simulink model "model_VS_PSH"  (R2020b)
settings: Solver=ode1  StartTime=0.0  StopTime=60  RelTol=1e-3
InitFcn:
  | xInitial = init_power_wind_dfig_det;
  | %Ts=5e-6;
values from neighbouring files (symbols this model uses):
  Cap_DClink = 20000e-6    (= 0.02)    [MAIN_VS_PSH.m]
  Efficiency = 0.9    [MAIN_VS_PSH.m]
  Fnom = 60    [MAIN_VS_PSH.m]
  H = 2.7    [MAIN_VS_PSH.m]
  Initial_Head = 1    [MAIN_VS_PSH.m]
  Initial_SOC = 0.8    [MAIN_VS_PSH.m]
  kmVdc = 20e3    (= 20000)    [MAIN_VS_PSH.m]
  Kp = 1    [MAIN_VS_PSH.m]
  kp_pll = 0.236583    [MAIN_T_PSH_IEEE39.m]    (also in MAIN_VS_PSH.m)
  Kpg = 1.3466e-5    (= 1.3466e-05)    [MAIN_VS_PSH.m]
  Kpr = 4.559e-5    (= 4.559e-05)    [MAIN_VS_PSH.m]
  Kvp = 6.1584    [MAIN_VS_PSH.m]
  Lm = Lb*Lmpu    [MAIN_VS_PSH.m]
  Lph = 3e-4    (= 0.0003)    [MAIN_VS_PSH.m]
  Lr = Lb*Lrpu    [MAIN_VS_PSH.m]
  Lrleakpu = 0.11    [MAIN_VS_PSH.m]
  Ls = Lb*Lspu    [MAIN_VS_PSH.m]
  Lsleakpu = 0.102    [MAIN_VS_PSH.m]
  Max_discharge_hrs = 10    [MAIN_VS_PSH.m]
  Mode = 0    [MAIN_FS_PSH_IEEE39.m]    (also in MAIN_VS_PSH.m = 1; plots_FS_PSH_IEEE39.m = 1; plots_VS_PSH.m = 1)
  Pnom = Srated*1e6    (= 300000000)    [MAIN_VS_PSH.m]
  Pref = 0.9    [MAIN_T_PSH_IEEE39.m]    (also in MAIN_VS_PSH.m = 1)
  QnL = 0    [MAIN_VS_PSH.m]
  Qref = 0    [MAIN_VS_PSH.m]
  Rrpu = 0.00607    [MAIN_VS_PSH.m]
  Rspu = 0.0054    [MAIN_VS_PSH.m]
  sigma = 1- Lmpu*Lmpu/(Lrpu^2)    (= 0.0485899542692)    [MAIN_VS_PSH.m]
  Srated = 300    [MAIN_VS_PSH.m]
  t_sw_off = 220    [MAIN_FS_PSH_IEEE39.m]    (also in MAIN_T_PSH_IEEE39.m; MAIN_VS_PSH.m = 45)
  t_sw_on = 130    [MAIN_FS_PSH_IEEE39.m]    (also in MAIN_T_PSH_IEEE39.m; MAIN_VS_PSH.m = 35)
  Ti = 0.01    [MAIN_VS_PSH.m]
  ti_pll = 0.0224242    [MAIN_T_PSH_IEEE39.m]    (also in MAIN_VS_PSH.m)
  Tig = 59.0944    [MAIN_VS_PSH.m]
  Tir = 197.953    [MAIN_VS_PSH.m]
  Ts = 25e-6    (= 2.5e-05)    [MAIN_FS_PSH_IEEE39.m]    (also in MAIN_T_PSH_IEEE39.m; MAIN_VS_PSH.m = 1e-07)
  TurnsRatio = 0.37912    [MAIN_VS_PSH.m]
  Tvi = 0.0013532    [MAIN_VS_PSH.m]
  V1 = sqrt(2)*Vnom_grid/sqrt(3)    [MAIN_VS_PSH.m]
  Vdc_ref = 40e3    (= 40000)    [MAIN_VS_PSH.m]
  Vnom_grid = 18e3    (= 18000)    [MAIN_VS_PSH.m]
  W1 = 2*pi*Fnom    (= 376.991118431)    [MAIN_VS_PSH.m]
  Xph = Lph*W1    (= 0.113097335529)    [MAIN_VS_PSH.m]
undefined symbols (not defined in the file or in its folder): magnitude
libraries: powerlib x49, powerlib_meascontrol x21, pid_lib x10, simulink_extras x4, simulink x1
(part 1 of 3)
settings Model: FPTRunName=Active  SimulationMode=accelerator  ExtModeAutoUpdateStatusClock=off  Creator=MathWorks  LastModifiedBy=mjimene
settings DataIOCC: MaxDataPoints=1500  SaveFormat=StructureWithTime  SignalLoggingSaveFormat=ModelDataLogs  SaveOutput=off  SignalLogging=off  DSMLogging=off  SaveTime=off
settings OptimizationCC: ExpressionDepthLimit=2147483647  InitFltsAndDblsToZero=on  LifeSpan=inf
settings DebuggingCC: SaveWithParameterizedLinksMsg=none  UnderspecifiedInitializationDetection=Classic  MergeDetectMultiDrivingBlocksExec=none  SignalResolutionControl=TryResolveAllWithWarning  SolverPrmCheckMsg=warning  FcnCallInpInsideContextMsg=warning  UnconnectedLineMsg=none  StateNameClashWarn=warning  SFUnexpectedBacktrackingDiag=warning  SFNoUnconditionalDefaultTransitionDiag=warning  SFExecutionAtInitializationDiag=none  ArithmeticOperatorsInVariantConditions=warning
settings HardwareCC: ProdBitPerPointer=32  ProdBitPerSizeT=32  ProdBitPerPtrDiffT=32  ProdLargestAtomicFloat=None  ProdIntDivRoundTo=Undefined  ProdEndianess=Unspecified  ProdWordSize=32  ProdHWDeviceType=32-bit Generic
settings ModelReferenceCC: PropagateSignalLabelsOutOfModel=off
settings SFSimCC: SimUseLocalCustomCode=off  CustomCodeUndefinedFunction=UseInterfaceOnly
settings RTWCC: RTWUseLocalCustomCode=off
settings CodeAppCC: StateflowObjectComments=on
settings GRTTargetCC: TargetFcnLib=ansi_tfl_tmw.mat  TargetLangStandard=C89/C90 (ANSI)  CombineOutputUpdateFcns=off  GRTInterface=on
settings ConfigComp: CovMetricSettings=dw  CovSaveCumulativeToWorkspaceVar=on  CovSaveSingleToWorkspaceVar=on  CovExternalEMLEnable=off  CovSFcnEnable=off
settings SimscapeCC: SimscapeNormalizeSystem=off

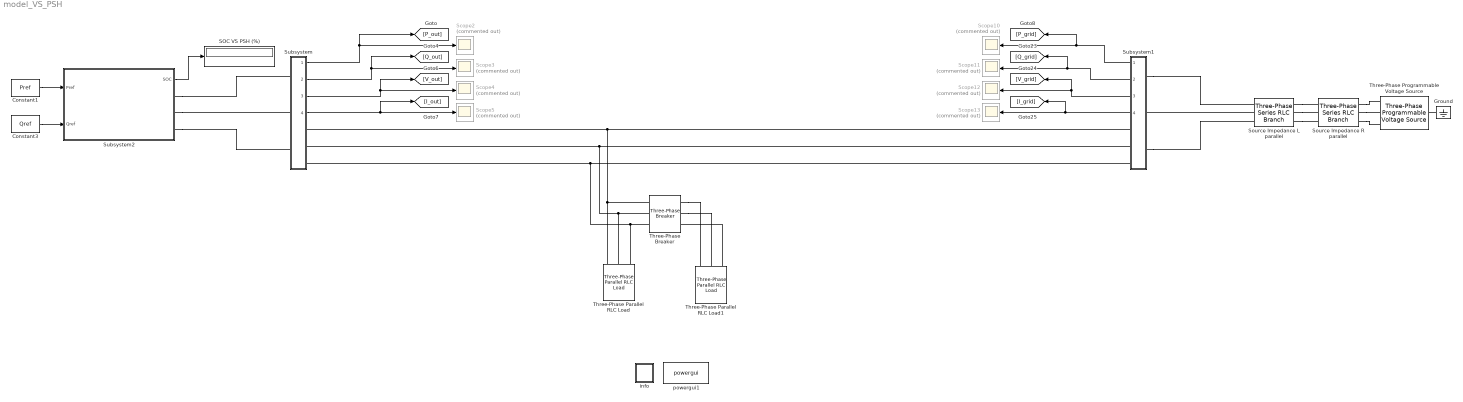
== system model_VS_PSH ==
  Constant1 : Constant  Value=Pref
  Constant3 : Constant  Value=Qref
  Ground : powerlib/Elements/Ground  LConnTagsString=a
  SOC VS PSH (%) : Display
  Scope{2..5,10..13} (8 alike) : Scope  Commented=on
  Source Impedance R parallel : powerlib/Elements/Three-Phase Series RLC Branch  LConnTagsString=A|B|C  RConnTagsString=A|B|C  BranchType=R  Resistance=0.0945*0.1/490  Inductance=0.01  Capacitance=[]  Measurements=None
  Source Impedance L parallel : powerlib/Elements/Three-Phase Series RLC Branch  LConnTagsString=A|B|C  RConnTagsString=A|B|C  BranchType=L  Resistance=1  Inductance=14.2e-4/490  Capacitance=[]  Measurements=None
  Subsystem : Subsystem
  Subsystem1 : Subsystem
  Subsystem2 : Subsystem
  Three-Phase Parallel RLC Load : powerlib/Elements/Three-Phase Parallel RLC Load  LConnTagsString=A|B|C  Configuration=Y (grounded)  NominalVoltage=18e3  Vabc=[1e3 1e3 1e3]  Vabcp=[1e3 1e3 1e3]  NominalFrequency=60  UnbalancedPower=off  ActivePower=50e6  InductivePower=0  CapacitivePower=0  Pabc=[10e3 9e3 11e3]  QLabc=[100 90 110]  QCabc=[100 90 110]  Pabcp=[10e3 9e3 11e3]  QLabcp=[100 90 110]  QCabcp=[100 90 110]  Measurements=None  LoadType=constant Z
  Three-Phase Parallel RLC Load1 : powerlib/Elements/Three-Phase Parallel RLC Load  LConnTagsString=A|B|C  Configuration=Y (grounded)  NominalVoltage=18e3  Vabc=[1e3 1e3 1e3]  Vabcp=[1e3 1e3 1e3]  NominalFrequency=60  UnbalancedPower=off  ActivePower=50e6  InductivePower=0  CapacitivePower=0  Pabc=[10e3 9e3 11e3]  QLabc=[100 90 110]  QCabc=[100 90 110]  Pabcp=[10e3 9e3 11e3]  QLabcp=[100 90 110]  QCabcp=[100 90 110]  Measurements=None  LoadType=constant Z
  Three-Phase Programmable Voltage Source : powerlib/Electrical Sources/Three-Phase Programmable Voltage Source  PositiveSequence=[18e3 0 60]  VariationEntity=None  VariationType=Table of time-amplitude pairs  VariationTypeAlt=Step  VariationStep=-0.5  VariationRate=10  VariationMagnitude=0.3  VariationFrequency=2  VariationTiming=[30 37]  VariationPhaseA=off  Amplitudes=[1 0.8 1.2 1.0]  TimeValues=[0 0.1 0.15 0.2]  HarmonicGeneration=off  HarmonicA=[3 0.2 -25 0]  HarmonicB=[2 0.15 35 2]  Timing="[0.05  3]"  BusType=swing  Pref=0  Qref=0  Qmin=-inf  Qmax=inf
  Three-Phase Breaker : powerlib/Elements/Three-Phase Breaker  InitialState=open  SwitchA=on  SwitchB=on  SwitchC=on  SwitchTimes=[t_sw_on t_sw_off]  External=off  BreakerResistance=0.01  SnubberResistance=1e6  SnubberCapacitance=inf  Measurements=None
  info : Subsystem
      settings: OpenFcn=showdemo(bdroot(gcb))
      mask Display: disp('?')
  powergui1 : powerlib/powergui  Priority=1  SimulationMode=Discrete  SampleTime=Ts  frequency=60  Iterations=50  frequencyindice=0  Pbase=100e6  ErrMax=1e-4  UnitsV=kV  UnitsW=MW  buscounter=0  FunctionMessages=off  echomessages=off  EnableUseOfTLC=off  CurrentSourceSwitches=off  DisableSnubberDevices=off  DisableRonSwitches=off  DisableVfSwitches=off  DisplayEquations=off  AutomaticDiscreteSolvers=off  SolverType=Tustin/Backward Euler (TBE)  Interpol=off  ExternalGateDelay=off  methode=off  Ts=100  x0status=blocks  SPID=on  SwTol=0  HookPort=off  NonlinearTolerance=1e-4  nMaxIteration=100  ContinueOnMaxIteration=off  RestoreLinks=warning  ResistiveCurrentMeasurement=off  Frange=[0:2:500]  Ylog=off  Xlog=on  ShowGrid=off  save=off  variable=ZData  structure=0  ZoomFFT=off  StartTime=0.0  cycles=1  DisplayStyle=1  fundamental=60  FreqAxis=off  MaxFrequency=1000  frequencyindicesteady=1  RmsSteady=1  display=off
  wires:
  Subsystem/1(Out1) -> [P_out], Scope2/1
  Subsystem/2(Out2) -> [Q_out], Scope3/1
  Subsystem/3(Out3) -> [V_out], Scope4/1
  Subsystem/4(Out4) -> [I_out], Scope5/1
  Subsystem1/4(Out4) -> [I_grid], Scope13/1
  Subsystem1/3(Out3) -> [V_grid], Scope12/1
  Subsystem1/2(Out2) -> [Q_grid], Scope11/1
  Subsystem1/1(Out1) -> [P_grid], Scope10/1
  Constant1/1 -> Subsystem2/1(Pref)
  Constant3/1 -> Subsystem2/2(Qref)
  Subsystem2/1(SOC) -> SOC VS PSH (%)/1
  connections:
  Three-Phase Parallel RLC Load1/LConn3 -- Three-Phase Breaker/RConn3
  Three-Phase Breaker/RConn2 -- Three-Phase Parallel RLC Load1/LConn2
  Three-Phase Breaker/RConn1 -- Three-Phase Parallel RLC Load1/LConn1
  Subsystem/RConn1 -- Three-Phase Parallel RLC Load/LConn1 -- Three-Phase Breaker/LConn1 -- Subsystem1/RConn1
  Subsystem1/RConn2 -- Three-Phase Parallel RLC Load/LConn2 -- Three-Phase Breaker/LConn2 -- Subsystem/RConn2
  Three-Phase Parallel RLC Load/LConn3 -- Three-Phase Breaker/LConn3 -- Subsystem1/RConn3 -- Subsystem/RConn3
  Subsystem2/RConn1 -- Subsystem/LConn1
  Subsystem2/RConn2 -- Subsystem/LConn2
  Subsystem2/RConn3 -- Subsystem/LConn3
  Subsystem1/LConn1 -- Source Impedance L parallel/LConn1
  Source Impedance L parallel/LConn2 -- Subsystem1/LConn2
  Subsystem1/LConn3 -- Source Impedance L parallel/LConn3
  Ground/LConn1 -- Three-Phase Programmable Voltage Source/LConn1
  Source Impedance L parallel/RConn1 -- Source Impedance R parallel/LConn1
  Source Impedance L parallel/RConn2 -- Source Impedance R parallel/LConn2
  Source Impedance L parallel/RConn3 -- Source Impedance R parallel/LConn3
  Source Impedance R parallel/RConn1 -- Three-Phase Programmable Voltage Source/RConn1
  Source Impedance R parallel/RConn2 -- Three-Phase Programmable Voltage Source/RConn2
  Source Impedance R parallel/RConn3 -- Three-Phase Programmable Voltage Source/RConn3

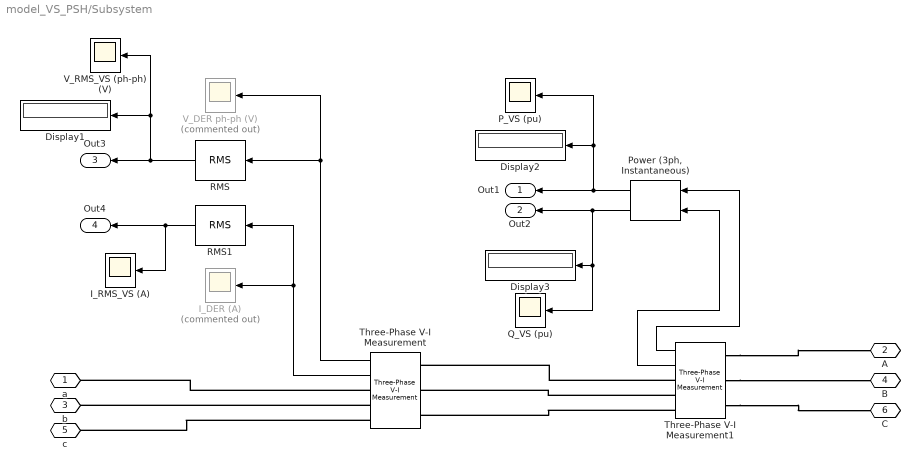
== system model_VS_PSH/Subsystem ==
  Display1 : Display
  Display2 : Display
  Display3 : Display
  I_DER (A) : Scope  Commented=on
  I_RMS_VS (A) : Scope
  P_VS (pu) : Scope
  "Power (3ph, Instantaneous)" : powerlib_meascontrol/Measurements/Power (3ph, Instantaneous)
  Q_VS (pu) : Scope
  RMS : powerlib_meascontrol/Measurements/RMS  TrueRMS=off  Freq=60  RMSInit=1  Ts=Ts
  RMS1 : powerlib_meascontrol/Measurements/RMS  TrueRMS=off  Freq=60  RMSInit=1  Ts=Ts
  Three-Phase V-I Measurement : powerlib/Measurements/Three-Phase V-I Measurement  VoltageMeasurement=phase-to-phase  SetLabelV=off  LabelV=Vabc  Vpu=off  VpuLL=off  CurrentMeasurement=yes  SetLabelI=off  LabelI=Iabc  Ipu=off  Pbase=100e6  Vbase=500e3  OutputType=Complex  PhasorSimulation=off  PSBequivalent=0
  Three-Phase V-I Measurement1 : powerlib/Measurements/Three-Phase V-I Measurement  VoltageMeasurement=phase-to-ground  SetLabelV=off  LabelV=Vabc  Vpu=off  VpuLL=off  CurrentMeasurement=yes  SetLabelI=off  LabelI=Iabc  Ipu=off  Pbase=100e6  Vbase=500e3  OutputType=Complex  PhasorSimulation=off  PSBequivalent=0
  V_DER ph-ph (V) : Scope  Commented=on
  V_RMS_VS (ph-ph) (V) : Scope
  a : PMIOPort  Side=Right
  A : PMIOPort  Port=2  Side=Left
  b : PMIOPort  Port=3  Side=Right
  B : PMIOPort  Port=4  Side=Left
  c : PMIOPort  Port=5  Side=Right
  C : PMIOPort  Port=6  Side=Left
  Out1 : Outport
  Out2 : Outport  Port=2
  Out3 : Outport  Port=3
  Out4 : Outport  Port=4
  wires:
  Three-Phase V-I Measurement1/1 -> "Power (3ph, Instantaneous)"/1
  Three-Phase V-I Measurement/1 -> RMS/1, V_DER ph-ph (V)/1
  Three-Phase V-I Measurement/2 -> RMS1/1, I_DER (A)/1
  RMS1/1 -> Out4/1, I_RMS_VS (A)/1
  Three-Phase V-I Measurement1/2 -> "Power (3ph, Instantaneous)"/2
  RMS/1 -> Out3/1, V_RMS_VS (ph-ph) (V)/1, Display1/1
  "Power (3ph, Instantaneous)"/1 -> Display2/1, P_VS (pu)/1, Out1/1
  "Power (3ph, Instantaneous)"/2 -> Q_VS (pu)/1, Display3/1, Out2/1
  connections:
  Three-Phase V-I Measurement1/RConn1 -- Three-Phase V-I Measurement/LConn1
  Three-Phase V-I Measurement1/RConn2 -- Three-Phase V-I Measurement/LConn2
  Three-Phase V-I Measurement1/RConn3 -- Three-Phase V-I Measurement/LConn3
  Three-Phase V-I Measurement/RConn2 -- b/RConn1
  Three-Phase V-I Measurement/RConn3 -- c/RConn1
  Three-Phase V-I Measurement1/LConn1 -- A/RConn1
  Three-Phase V-I Measurement/RConn1 -- a/RConn1
  Three-Phase V-I Measurement1/LConn2 -- B/RConn1
  Three-Phase V-I Measurement1/LConn3 -- C/RConn1

== system model_VS_PSH/Subsystem1 ==
  "Power (3ph, Instantaneous)" : powerlib_meascontrol/Measurements/Power (3ph, Instantaneous)
  Three-Phase V-I Measurement : powerlib/Measurements/Three-Phase V-I Measurement  VoltageMeasurement=phase-to-phase  SetLabelV=off  LabelV=Vabc  Vpu=off  VpuLL=off  CurrentMeasurement=yes  SetLabelI=off  LabelI=Iabc  Ipu=off  Pbase=100e6  Vbase=500e3  OutputType=Complex  PhasorSimulation=off  PSBequivalent=0
  Three-Phase V-I Measurement1 : powerlib/Measurements/Three-Phase V-I Measurement  VoltageMeasurement=phase-to-ground  SetLabelV=off  LabelV=Vabc  Vpu=off  VpuLL=off  CurrentMeasurement=yes  SetLabelI=off  LabelI=Iabc  Ipu=off  Pbase=100e6  Vbase=500e3  OutputType=Complex  PhasorSimulation=off  PSBequivalent=0
  a : PMIOPort  Side=Right
  A : PMIOPort  Port=2  Side=Left
  b : PMIOPort  Port=3  Side=Right
  B : PMIOPort  Port=4  Side=Left
  c : PMIOPort  Port=5  Side=Right
  C : PMIOPort  Port=6  Side=Left
  Out1 : Outport
  Out2 : Outport  Port=2
  Out3 : Outport  Port=3
  Out4 : Outport  Port=4
  wires:
  Three-Phase V-I Measurement1/1 -> "Power (3ph, Instantaneous)"/1
  Three-Phase V-I Measurement/2 -> Out4/1
  Three-Phase V-I Measurement1/2 -> "Power (3ph, Instantaneous)"/2
  Three-Phase V-I Measurement/1 -> Out3/1
  "Power (3ph, Instantaneous)"/1 -> Out1/1
  "Power (3ph, Instantaneous)"/2 -> Out2/1
  connections:
  Three-Phase V-I Measurement1/RConn1 -- Three-Phase V-I Measurement/LConn1
  Three-Phase V-I Measurement1/RConn2 -- Three-Phase V-I Measurement/LConn2
  Three-Phase V-I Measurement1/RConn3 -- Three-Phase V-I Measurement/LConn3
  Three-Phase V-I Measurement/RConn2 -- b/RConn1
  Three-Phase V-I Measurement/RConn3 -- c/RConn1
  Three-Phase V-I Measurement1/LConn1 -- A/RConn1
  Three-Phase V-I Measurement/RConn1 -- a/RConn1
  Three-Phase V-I Measurement1/LConn2 -- B/RConn1
  Three-Phase V-I Measurement1/LConn3 -- C/RConn1

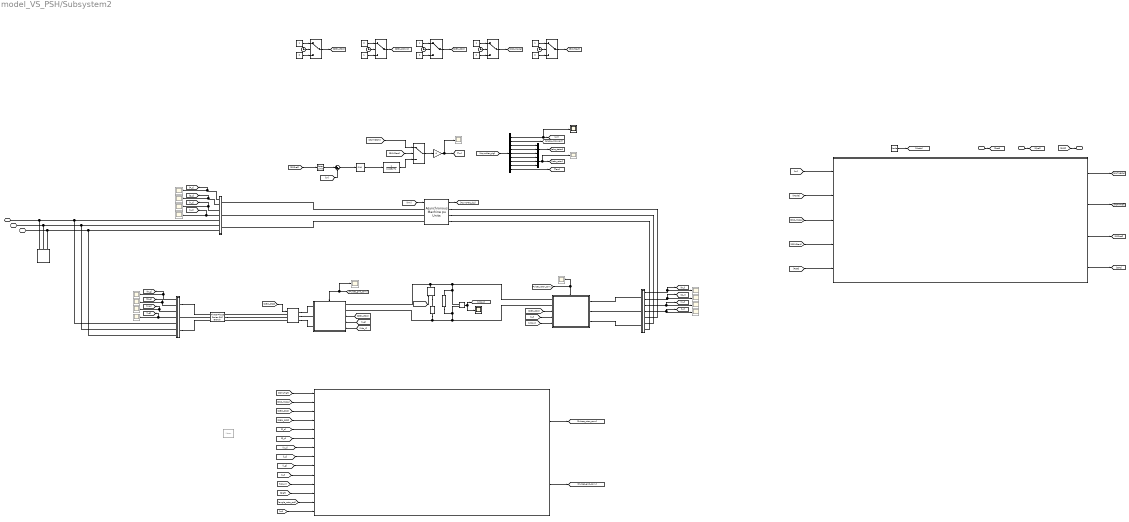
== system model_VS_PSH/Subsystem2 ==
  note: AC-DC-AC Converter
      | Average Model
  note: GSC measurements
  note: Variable Speed Hydro PSH
  note: RSC measurements
  note: Wound-Rotor
      | Induction Generator
  note: Measurement and controls
  note: Intialization sequence
  Pref : Inport
  Qref : Inport  Port=2
  Asynchronous Machine pu Units : powerlib/Machines/Asynchronous Machine pu Units  RotorType=Wound  PresetModel=No  MechanicalLoad=Torque Tm  ShowDetailedParameters=on  ReferenceFrame=Rotor  Units=pu  MeasurementBus=off  NominalParameters=[ Pnom Vnom_grid Fnom ]  Stator=[ Rspu Lsleakpu]  Rotor=[ Rrpu Lrleakpu]  Cage1=[0.01909 0.0397]  Cage2=[0.01909 0.0397]  Lm=Lmpu  Mechanical=[H 0.01 1]  PolePairs=3  InitialConditions=[0, pi, 0,0,0, 0,-120,120, 0,0,0, 0,-120, 120]  SimulateSaturation=off  Saturation="[0.212,0.4201,0.8125,1.0979,1.4799,2.2457,3.2586,4.5763,6.4763 ;   0.5,0.7,0.9,1,1.1,1.2 ,1.3,1.4,1.5]"  LoadFlowParameters=0  TsPowergui=0  TsBlock=-1  IterativeModel=Trapezoidal non iterative  IterativeDiscreteModel=Trapezoidal non iterative  Pmec=0
      settings: SourceProductBaseCode=PS
  Breaker1 : powerlib/Elements/Breaker  InitialState=1  SwitchingTimes="[1/60  5/60]"  External=on  BreakerResistance=0.01  SnubberResistance=1e6  SnubberCapacitance=inf  Measurements=None  MoreParameters=on  NoBreakLoop=off
  Bus Selector : BusSelector  OutputSignals=Mechanical.Rotor speed (wm),Mechanical.Rotor angle thetam (rad),Stator measurements.Stator current is_a (pu),Stator measurements.Stator current is_b (pu),Stator measurements.Stator current is_c (pu),Rotor measurements.Rotor current ir_a (pu),Rotor measurements.Rotor current ir_b (pu),Rotor measurements.Rotor current ir_c (pu),Mechanical.Electromagnetic torque Te (pu)
  Clock{1..5} (5 alike) : Clock
  Constant1 : Constant  Value=Mode
  Constant{6..8,10..11} (5 alike) : Constant
  Constant{2..5,9} (5 alike) : Constant  Value=0
  DC Voltage Source : powerlib/Electrical Sources/DC Voltage Source  Amplitude=40e3  Measurements=None
  Discrete PID Controller : pid_lib/PID Controller  Controller=PI  Form=Parallel  TimeDomain=Continuous-time  UseExternalTs=off  SampleTime=-1  IntegratorMethod=Forward Euler  FilterMethod=Forward Euler  ControllerParametersSource=internal  P=10  I=1  D=0  UseFilter=on  N=100  TunerSelectOption=Transfer Function Based (PID Tuner App)  InitialConditionSource=internal  InitialConditionForIntegrator=0  InitialConditionForFilter=0  DifferentiatorICPrevScaledInput=0  ExternalReset=none  TrackingMode=off  Kt=1  LimitOutput=on  SatLimitsSource=internal  UpperSaturationLimit=1  LowerSaturationLimit=-1  LinearizeAsGain=off  AntiWindupMode=back-calculation  Kb=1  POutMin=[]  POutMax=[]  IOutMin=[]  IOutMax=[]  DOutMin=[]  DOutMax=[]  NOutMin=[]  NOutMax=[]  SumOutMin=[]  SumOutMax=[]  SaturationOutMin=[]  SaturationOutMax=[]  PParamMin=[]  PParamMax=[]  IParamMin=[]  IParamMax=[]  DParamMin=[]  DParamMax=[]  NParamMin=[]  NParamMax=[]  KbParamMin=[]  KbParamMax=[]  KtParamMin=[]  KtParamMax=[]  KbOutMin=[]  KbOutMax=[]  KtOutMin=[]  KtOutMax=[]  IntegratorOutMin=[]  IntegratorOutMax=[]  FilterOutMin=[]  FilterOutMax=[]  SumI1OutMin=[]  SumI1OutMax=[]  SumI2OutMin=[]  SumI2OutMax=[]  SumI3OutMin=[]  SumI3OutMax=[]  SumI4OutMin=[]  SumI4OutMax=[]  SumDOutMin=[]  SumDOutMax=[]  DifferentiatorOutMin=[]  DifferentiatorOutMax=[]  FilterDiffOutCoefMin=[]  FilterDiffOutCoefMax=[]  ReciprocalOutMin=[]  ReciprocalOutMax=[]  SumDenOutMin=[]  SumDenOutMax=[]  SumNumOutMin=[]  SumNumOutMax=[]  DivideOutMin=[]  DivideOutMax=[]  UdiffTsProdOutMin=[]  UdiffTsProdOutMax=[]  NTsProdOutMin=[]  NTsProdOutMax=[]  UintegralTsProdOutMin=[]  UintegralTsProdOutMax=[]  UngainTsProdOutMin=[]  UngainTsProdOutMax=[]  IntegratorContinuousStateAttributes=''  IntegratorStateMustResolveToSignalObject=off  IntegratorRTWStateStorageClass=Auto  FilterContinuousStateAttributes=''  FilterStateMustResolveToSignalObject=off  FilterRTWStateStorageClass=Auto  ParallelPVariant=InternalParameters  IdealPVariant=Disabled  IVariant=InternalParameters  DVariant=Disabled  IntegratorVariant=Continuous  SatVariant=Enabled  AWVariant=BackCalculation  PCopyVariant=Disabled  TRVariant=Disabled  FdbkBlocksVariant=Forward  IdealPFdbkVariant=Disabled  SatFdbkVariant=Disabled  DerivativeFilterVariant=Disabled  NVariant=Disabled  NCopyVariant=Disabled_SignalSpec  FilterICVariant=Disabled  IntegratorICVariant=InternalICs  ExternalResetVariant=Disabled  TRSumVariant=Passthrough  SumFdbkVariant=Disabled  SumVariant=Sum_PI  TsampFilterVariant=InternalTs  TsampNgainVariant=Passthrough  TsampIntegralVariant=Passthrough  ExternalSaturationOutDataTypeStr=Inherit: Same as second input
  Gain1 : Gain  Gain=-1
  Mean : powerlib_meascontrol/Measurements/Mean  Commented=on  Freq=60  Vinit=0  Ts=Ts
  Mux : Mux  Inputs=3
  Mux1 : Mux  Inputs=3
  Rate Limiter : RateLimiter  RisingSlewLimit=0.1  FallingSlewLimit=-0.1  SampleTimeMode=inherited
  Scope{2,5..6,8,10..13,15,17..22} (15 alike) : Scope  Commented=on
  Scope16 : Scope
  Series RLC Branch : powerlib/Elements/Series RLC Branch  LConnTagsString=__new0  RConnTagsString=__new0  BranchType=RC  Resistance=0.07  Inductance=1e-3  SetiL0=off  InitialCurrent=0  Capacitance=Cap_DClink  Setx0=on  InitialVoltage=Vdc_ref  Measurements=Branch voltage
  Subsystem : Subsystem
  Subsystem1 : Subsystem
  Subsystem2 : Subsystem
  Subsystem3 : Subsystem
  Subsystem4 : Subsystem
      settings: PortSchema="{\"entries\":[{\"content\":{\"sides\":[{\"content\":{\"connectorIds\":[\"LConn1\",\"LConn2\",\"LConn3\"]},\"type\":\"ConnectorPlacement.EquallySpacedRectSide\",\"uuid\":\"94841cf4-93b3-4880-baa1-84da98f5225b\"},{\"content\":{\"connectorIds\":[\"In2\",\"In3\",\"In4\",\"RConn1\",\"RConn2\"],\"side\":\"RIGHT\"},\"type\":\"ConnectorPlacement.EquallySpacedRectSide\",\"uuid\":\"b88fbc7b-9829-4cc6-9f20-4a6a61ae3277\"},{\"content\":{\"connectorIds\":[],\"side\":\"TOP\"},\"type\":\"ConnectorPlacement.EquallySpacedRectSide\",\"uuid\":\"f514aa96-3bbf-42de-9cc7-b6fe6a85c8a9\"},{\"content\":{\"connectorIds\":[\"In1\"],\"side\":\"BOTTOM\"},\"type\":\"ConnectorPlacement.EquallySpacedRectSide\",\"uuid\":\"3681cdf3-8976-49a1-89c5-977238c808bf\"},{\"content\":{\"connectorIds\":[],\"side\":\"HIDDEN\"},\"type\":\"ConnectorPlacement.EquallySpacedRectSide\",\"uuid\":\"6f5fb23e-3fe6-44f2-8b50-581ba0dee18c\"}]},\"type\":\"ConnectorPlacement.EquallySpacedConnector\",\"uuid\":\"eff892e2-74e2-4cdd-8af6-0e483dd06ee4\"}],\"packageUris\":[\"http://schema.mathworks.com/mf0/Connector/R2020b\"],\"version\":\"1.0\"}"
  Subsystem5 : Subsystem
  Subsystem6 : Subsystem
      settings: PortSchema="{\"entries\":[{\"content\":{\"sides\":[{\"content\":{\"connectorIds\":[\"LConn1\",\"LConn2\",\"LConn3\"]},\"type\":\"ConnectorPlacement.EquallySpacedRectSide\",\"uuid\":\"94841cf4-93b3-4880-baa1-84da98f5225b\"},{\"content\":{\"connectorIds\":[\"In2\",\"In3\",\"In4\",\"RConn1\",\"RConn2\"],\"side\":\"RIGHT\"},\"type\":\"ConnectorPlacement.EquallySpacedRectSide\",\"uuid\":\"b88fbc7b-9829-4cc6-9f20-4a6a61ae3277\"},{\"content\":{\"connectorIds\":[],\"side\":\"TOP\"},\"type\":\"ConnectorPlacement.EquallySpacedRectSide\",\"uuid\":\"f514aa96-3bbf-42de-9cc7-b6fe6a85c8a9\"},{\"content\":{\"connectorIds\":[\"In1\"],\"side\":\"BOTTOM\"},\"type\":\"ConnectorPlacement.EquallySpacedRectSide\",\"uuid\":\"3681cdf3-8976-49a1-89c5-977238c808bf\"},{\"content\":{\"connectorIds\":[],\"side\":\"HIDDEN\"},\"type\":\"ConnectorPlacement.EquallySpacedRectSide\",\"uuid\":\"6f5fb23e-3fe6-44f2-8b50-581ba0dee18c\"}]},\"type\":\"ConnectorPlacement.EquallySpacedConnector\",\"uuid\":\"eff892e2-74e2-4cdd-8af6-0e483dd06ee4\"}],\"packageUris\":[\"http://schema.mathworks.com/mf0/Connector/R2020b\"],\"version\":\"1.0\"}"
  Sum : Sum  Inputs=|+-
  Switch1 : Switch  Criteria=u2 > Threshold  Threshold=10
  Switch14 : Switch  Threshold=1
  Switch2 : Switch  Criteria=u2 > Threshold  Threshold=4
  Switch3 : Switch  Criteria=u2 > Threshold  Threshold=2
  Switch4 : Switch  Criteria=u2 > Threshold  Threshold=3
  Switch8 : Switch  Criteria=u2 > Threshold  Threshold=5
  Three-Phase Parallel RLC Load1 : powerlib/Elements/Three-Phase Parallel RLC Load  LConnTagsString=A|B|C  Configuration=Y (grounded)  NominalVoltage=Vnom_grid  Vabc=[1e3 1e3 1e3]  Vabcp=[1e3 1e3 1e3]  NominalFrequency=60  UnbalancedPower=off  ActivePower=10e3  InductivePower=0  CapacitivePower=0  Pabc=[10e3 9e3 11e3]  QLabc=[100 90 110]  QCabc=[100 90 110]  Pabcp=[10e3 9e3 11e3]  QLabcp=[100 90 110]  QCabcp=[100 90 110]  Measurements=None  LoadType=constant Z
  Three-Phase Series RLC Branch : powerlib/Elements/Three-Phase Series RLC Branch  LConnTagsString=A|B|C  RConnTagsString=A|B|C  BranchType=RL  Resistance=0.05  Inductance=Lph  Capacitance=1e-6  Measurements=None
  Three-Phase Breaker : powerlib/Elements/Three-Phase Breaker  InitialState=open  SwitchA=on  SwitchB=on  SwitchC=on  SwitchTimes="[1/60  5/60]"  External=on  BreakerResistance=0.0001  SnubberResistance=1e6  SnubberCapacitance=inf  Measurements=None
  Tm : Scope  Commented=on
  Transfer Fcn1 : TransferFcn  Denominator=[0.005 1]
  Vdc : Scope
  Voltage Measurement1 : powerlib/Measurements/Voltage Measurement  PhasorSimulation=off  OutputType=Complex  PSBequivalent=0
  A1 : PMIOPort  Tag=PMCPort  Side=Right
  B1 : PMIOPort  Tag=PMCPort  Port=2  Side=Right
  C1 : PMIOPort  Tag=PMCPort  Port=3  Side=Right
  SOC : Outport
  wires:
  Clock5/1 -> Switch4/2
  Gain1/1 -> [Tm], Tm/1
  [Tm] -> Asynchronous Machine pu Units/1
  Constant9/1 -> Switch3/3
  Subsystem1/2(Out2) -> [Q_s], Scope11/1
  Voltage Measurement1/1 -> Vdc/1, [Vdc_V]
  Pref/1 -> [Pset]
  Qref/1 -> [Qref]
  Switch3/1 -> [DBlk_GSC]
  Switch2/1 -> [DBlk_RSC]
  [DBlk_DClink] -> Breaker1/1
  Subsystem2/2(Out2) -> [Q_r], Scope20/1
  Constant3/1 -> Switch4/1
  Subsystem2/4(Out4) -> Scope18/1, [I_r]
  Constant11/1 -> Switch4/3
  [SOC] -> SOC/1
  Subsystem/4(SOC_out) -> [SOC]
  Bus Selector/6 -> Mux1/1  "<Rotor current ir_a (pu)>"
  Subsystem2/3(Out3) -> [V_r], Scope5/1
  Subsystem3/1(Out1) -> [P_g], Scope22/1
  [Pulses_grid_conv] -> Subsystem4/1(m), Scope2/1
  Bus Selector/8 -> Mux1/3  "<Rotor current ir_c (pu)>"
  [Pulses_rotor_conv] -> Subsystem6/1(m), Scope17/1
  [DBlk_GSC] -> Three-Phase Breaker/1
  Subsystem1/3(Out3) -> [V_s], Scope12/1
  [Vdc_V] -> Subsystem4/2(VdcLink)
  Subsystem/2(PSTATref) -> [PSTATref]
  Mux/1 -> [Iabc_stator]
  [DBlk_RSC] -> Subsystem6/4(DBlk_RSC)
  [Vdc_V] -> Subsystem6/2(VdcLink)
  [I_r] -> Subsystem6/3(Iabc)
  [Pset] -> Subsystem/5(Pset)
  [DBlk_GSC] -> Subsystem4/4(DBlk_GSC)
  Subsystem1/4(Out4) -> [I_s], Scope13/1
  [AsyncMac_sig] -> Bus Selector/1
  [SPDref] -> Rate Limiter/1
  Subsystem3/4(Out4) -> [I_g], Scope21/1
  Subsystem3/3(Out3) -> [V_g], Scope15/1
  Constant7/1 -> Switch1/1
  Subsystem1/1(Out1) -> [P_s], Scope10/1
  Subsystem3/2(Out2) -> [Q_g], Scope6/1
  Rate Limiter/1 -> Sum/1
  Constant1/1 -> [Mode]
  Bus Selector/9 -> [Tem]  "<Electromagnetic torque Te (pu)>"
  Clock4/1 -> Switch3/2
  Constant4/1 -> Switch1/3
  Bus Selector/5 -> Mux/3  "<Stator current is_c (pu)>"
  Switch1/1 -> [GOVStart]
  [G1TMECH] -> Switch14/1
  Subsystem/3(SPDref_out) -> [SPDref]
  Constant6/1 -> Switch8/1
  Clock2/1 -> Switch1/2
  Discrete PID Controller/1 -> Transfer Fcn1/1  "Id_ref"
  Clock1/1 -> Switch8/2
  [GOVStart] -> Switch14/2
  [wr] -> Sum/2
  Switch8/1 -> [RSC_Mode]
  [wr] -> Subsystem/1(wr)
  Bus Selector/1 -> Scope16/1, [wr]  "<Rotor speed (wm)>"
  [GOVStart] -> Subsystem/4(GOVStart)
  [Mode] -> Subsystem/2(TurbPump)
  Clock3/1 -> Switch2/2
  [RSC_Mode] -> Subsystem/3(RSC_Mode)
  Bus Selector/7 -> Mux1/2  "<Rotor current ir_b (pu)>"
  Switch14/1 -> Gain1/1
  Bus Selector/4 -> Mux/2  "<Stator current is_b (pu)>"
  Bus Selector/3 -> Mux/1  "<Stator current is_a (pu)>"
  Constant8/1 -> Switch2/1
  Subsystem/1(Tm_PSH) -> [G1TMECH]
  Mux1/1 -> Scope8/1, [Iabc_rotor]
  Sum/1 -> Discrete PID Controller/1
  Constant10/1 -> Switch3/1
  Asynchronous Machine pu Units/1 -> [AsyncMac_sig]
  [I_g] -> Subsystem4/3(Iabc)
  Transfer Fcn1/1 -> Switch14/3
  Switch4/1 -> [DBlk_DClink]
  Subsystem2/1(Out1) -> [P_r], Scope19/1
  Constant2/1 -> Switch8/3
  Bus Selector/2 -> [angle_rotor_rad]  "<Rotor angle thetam (rad)>"
  Constant5/1 -> Switch2/3
  [DBlk_GSC] -> Subsystem5/4(DBlk_GSC)
  [DBlk_RSC] -> Subsystem5/3(DBlk_RSC)
  [V_s] -> Subsystem5/7(V_s)
  [PSTATref] -> Subsystem5/1(PSTATref)
  [RSC_Mode] -> Subsystem5/2(RSC_Mode)
  [Qref] -> Subsystem5/12(Qref)
  [I_r] -> Subsystem5/10(I_r)
  [I_g] -> Subsystem5/9(I_g)
  [I_s] -> Subsystem5/8(I_s)
  [Vdc_V] -> Subsystem5/11(Vdc_V)
  [Q_s] -> Subsystem5/6(Q_s)
  [wr] -> Subsystem5/14(wr)
  [angle_rotor_rad] -> Subsystem5/13(angle_rotor_rad)
  Subsystem5/2(Pulses_grid_conv) -> [Pulses_grid_conv]
  Subsystem5/1(Pulses_rotor_conv) -> [Pulses_rotor_conv]
  [P_s] -> Subsystem5/5(P_s)
  connections:
  Voltage Measurement1/LConn1 -- Series RLC Branch/LConn1 -- Subsystem6/RConn2 -- Breaker1/RConn1 -- Subsystem4/RConn2
  Subsystem3/RConn2 -- Subsystem1/RConn2 -- Three-Phase Parallel RLC Load1/LConn2 -- B1/RConn1
  Series RLC Branch/RConn1 -- Voltage Measurement1/LConn2 -- Subsystem6/RConn1 -- DC Voltage Source/LConn1 -- Subsystem4/RConn1
  Subsystem3/RConn1 -- Three-Phase Parallel RLC Load1/LConn1 -- A1/RConn1 -- Subsystem1/RConn1
  Subsystem3/RConn3 -- Subsystem1/RConn3 -- Three-Phase Parallel RLC Load1/LConn3 -- C1/RConn1
  Subsystem6/LConn1 -- Subsystem2/LConn3
  Asynchronous Machine pu Units/RConn3 -- Subsystem2/RConn3
  Asynchronous Machine pu Units/LConn1 -- Subsystem1/LConn1
  Asynchronous Machine pu Units/LConn2 -- Subsystem1/LConn2
  Asynchronous Machine pu Units/LConn3 -- Subsystem1/LConn3
  Breaker1/LConn1 -- DC Voltage Source/RConn1
  Three-Phase Breaker/RConn1 -- Subsystem4/LConn3
  Three-Phase Breaker/RConn3 -- Subsystem4/LConn1
  Subsystem6/LConn3 -- Subsystem2/LConn1
  Three-Phase Breaker/RConn2 -- Subsystem4/LConn2
  Subsystem3/LConn3 -- Three-Phase Series RLC Branch/LConn3
  Three-Phase Breaker/LConn3 -- Three-Phase Series RLC Branch/RConn3
  Subsystem3/LConn1 -- Three-Phase Series RLC Branch/LConn1
  Subsystem6/LConn2 -- Subsystem2/LConn2
  Three-Phase Series RLC Branch/LConn2 -- Subsystem3/LConn2
  Three-Phase Series RLC Branch/RConn2 -- Three-Phase Breaker/LConn2
  Asynchronous Machine pu Units/RConn2 -- Subsystem2/RConn2
  Asynchronous Machine pu Units/RConn1 -- Subsystem2/RConn1
  Three-Phase Breaker/LConn1 -- Three-Phase Series RLC Branch/RConn1

== system model_VS_PSH/info ==

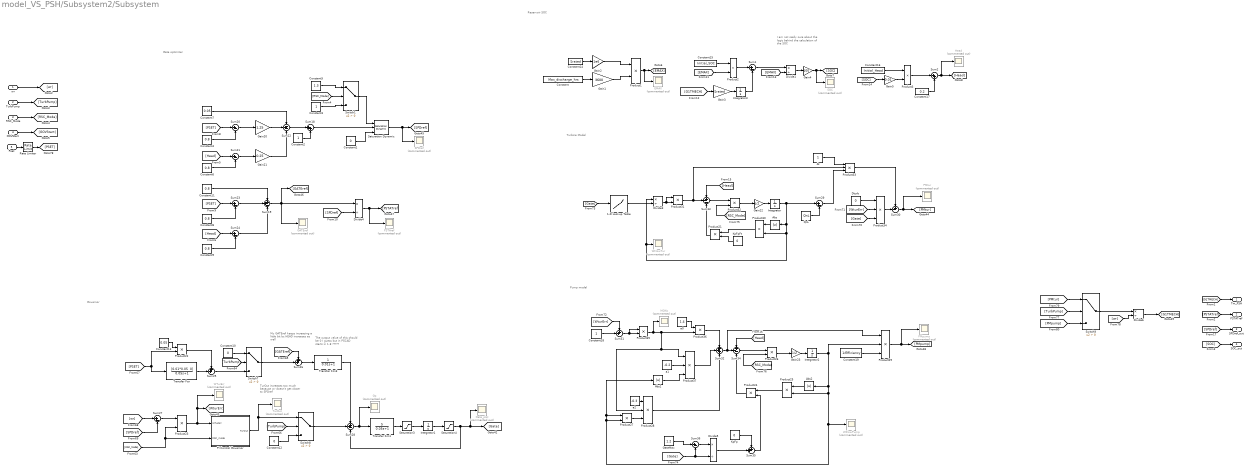
== system model_VS_PSH/Subsystem2/Subsystem ==
  note: Pump model
  note: Turbine Model
  note: Reservoir SOC
  note: Governor
  note: Gate optimizer
  note: The output value of this should be 0 I guess but in PSCAD starts in 1.8
      | ?????
  note: I am not really sure about the logic behind the calculation of the SOC
  note: TurOut increases too much because wr doesn't get closer to SPDref
  note: My GATEref keeps increasing a little bit bc HEAD increases as well
  wr : Inport
  TurbPump : Inport  Port=2
  RSC_Mode : Inport  Port=3
  GOVStart : Inport  Port=4
  Pset : Inport  Port=5
  1-D Lookup Table : Lookup_n-D  NumberOfTableDimensions=1  BreakpointsForDimension1=[0, 0.2, 0.4 , 0.6, 0.8, 1]  Table=[0, 0.2, 0.4 , 0.6, 0.8, 1]  InternalRulePriority=Speed  RndMeth=Simplest  InputSameDT=on
  Abs : Abs
  Abs1 : Abs
  Abs2 : Abs
  At : Constant
  Constant : Constant  Value=Max_discharge_hrs
  Constant1 : Constant  Value=0
  Constant10 : Constant  Value=0
  Constant{4,6,8..9,11} (5 alike) : Constant  Value=0.8
  Constant12 : Constant  Value=0
  Constant13 : Constant  Value=0.05
  Constant14 : Constant  Value=Srated
  Constant15 : Constant  Value=Initial_SOC
  Constant16 : Constant  Value=Initial_Head
  Constant17 : Constant  Value=0.2
  Constant18 : Constant
  Constant19 : Constant  Value=1/Efficiency
  Constant2 : Constant
  Constant3 : Constant
  Constant5 : Constant  Value=1.3
  Constant7 : Constant  Value=0.05
  Divide{1,3..6} (5 alike) : Product  Inputs=*/
  Dturb : Constant  Value=0
  EMAX : Scope  Commented=on
  GATEref : Scope  Commented=on
  Gain1 : Gain  Gain=3600
  Gain2 : Gain  Gain=1e6
  Gain20 : Gain  Gain=1.25
  Gain21 : Gain  Gain=0.25
  Gain22 : Gain  Gain=1/2
  Gain23 : Gain  Gain=1/2
  Gain3 : Gain  Gain=Srated
  Gain4 : Gain  Gain=100
  Gain5 : Gain  Gain=0.01
  GateMax : Constant  Value=1.2
  Gate_plot : Scope  Commented=on
  Gp : Scope  Commented=on
  Head : Scope  Commented=on
  Integrator : Integrator  InitialCondition=0.9068
  Integrator1 : Integrator
  Integrator2 : Integrator  InitialCondition=0.9068
  Integrator3 : Integrator  InitialCondition=0.9068
  KpFp : Constant  Value=0
  KpFpFt : Constant  Value=0
  MONx : Scope  Commented=on
  PI Control Governor : Subsystem
  PMpump : Scope  Commented=on
  PMtur : Scope  Commented=on
  PSTAref : Scope  Commented=on
  Product{1..3,21..27,30..32,35..36} (15 alike) : Product
  Product{28..29,33..34,37} (5 alike) : Product  Inputs=3
  QnL : Constant  Value=QnL
  Rate Limiter : RateLimiter  RisingSlewLimit=0.05  FallingSlewLimit=-0.05  SampleTimeMode=inherited  InitialCondition=1
  SOC : Scope  Commented=on
  SPDref : Scope  Commented=on
  Saturation Dynamic : simulink/Discontinuities/Saturation Dynamic  OutMin=[]  OutMax=[]  OutDataTypeStr=Inherit: Same as second input  OutDataType=fixdt(1, 16)  OutScaling=2^-10  DoSatur=off
  Saturation3 : Saturate  UpperLimit=0.1  LowerLimit=-0.1
  Saturation4 : Saturate  UpperLimit=1.2  LowerLimit=0.075
  Sum{1,20..21,23..24,27,29,36} (8 alike) : Sum  Inputs=|+-
  Sum18 : Sum  Inputs=|++
  Sum19 : Sum  Inputs=++-
  Sum2 : Sum  Inputs=|++
  Sum22 : Sum  Inputs=-+-
  Sum{25..26,31,35} (4 alike) : Sum  Inputs=++|
  Sum28 : Sum  Inputs=+--
  Sum30 : Sum  Inputs=+-|
  Sum32 : Sum  Inputs=+++
  Sum33 : Sum  Inputs=+--
  Sum34 : Sum  Inputs=+--
  Switch{1,7..9} (4 alike) : Switch  Criteria=u2 > Threshold
  Transfer Fcn : TransferFcn  Numerator="[0.01*0.05  0]"  Denominator=[0.05 1]
  Transfer Fcn1 : TransferFcn  Numerator=[5]  Denominator=[0.05 1]
  Transfer Fcn3 : TransferFcn  Denominator=[0.01 1]
  TurOut : Scope  Commented=on
  WFlowPump : Scope  Commented=on
  WFlowTur : Scope  Commented=on
  WTurErr : Scope  Commented=on
  a0 : Constant  Value=1.4
  a1 : Constant  Value=-0.2
  a2 : Constant  Value=-0.3
  Tm_PSH : Outport
  PSTATref : Outport  Port=2
  SPDref_out : Outport  Port=3
  SOC_out : Outport  Port=4
  wires:
  [Head] -> Sum33/1
  [Head] -> Sum21/1
  [RSC_Mode] -> PI Control Governor/2(RSC_mode), Product23/2
  Sum20/1 -> Gain20/1
  Divide4/1 -> PSTAref/1, [PSTATref]
  Gain22/1 -> Integrator/1
  Transfer Fcn3/1 -> Sum28/1
  Sum22/1 -> Sum18/1
  Gain23/1 -> Integrator2/1
  [wr] -> Divide6/2
  Constant6/1 -> Sum21/2
  Rate Limiter/1 -> [PSET]
  Constant12/1 -> Switch8/3
  Sum30/1 -> PMtur/1, [PMtur]
  a1/1 -> Product37/2
  Sum18/1 -> Saturation Dynamic/2
  [GATEref] -> Sum26/1
  Product31/1 -> Product33/2, Sum33/2
  [RSC_Mode] -> Product26/2
  Sum21/1 -> Gain21/1
  Constant8/1 -> Sum23/2
  Sum28/1 -> Gp/1, Transfer Fcn1/1
  Pset/1 -> Rate Limiter/1
  Sum31/1 -> Product35/1, Product35/2
  Constant10/1 -> Switch7/1
  Constant7/1 -> Sum22/1
  Constant18/1 -> Sum31/2
  Dturb/1 -> Product34/1
  Product23/1 -> PI Control Governor/1(WTurErr), WTurErr/1, [WturErr]
  Sum23/1 -> Sum19/2
  Integrator2/1 -> Product29/2, Abs1/1, Product27/1, Product27/2, WFlowPump/1, Product25/2, Abs2/1
  [wr] -> Sum27/1
  Sum35/1 -> Product24/2
  Constant9/1 -> Sum24/2
  Constant2/1 -> Sum18/2
  [TurbPump] -> Switch9/2
  [PSET] -> Transfer Fcn/1, Product22/2
  [Gate] -> Sum36/2, Divide5/2
  1-D Lookup Table/1 -> Divide3/2
  Saturation4/1 -> Gate_plot/1, [Gate], Sum28/3
  Product29/1 -> PMpump/1, [PMpump]
  Product22/1 -> Sum25/1
  Integrator1/1 -> Saturation4/1
  [PMtur] -> Switch9/1
  Saturation3/1 -> Integrator1/1
  Sum26/1 -> Transfer Fcn3/1
  Gain20/1 -> Sum22/2
  [Gate] -> Product34/3
  Transfer Fcn/1 -> Sum25/2
  Product33/1 -> Sum30/1
  Sum33/1 -> Product32/1
  Product21/1 -> Sum33/3
  [SPDref] -> Sum27/2
  [TurbPump] -> Switch7/2
  [Head] -> Sum24/1
  Abs2/1 -> Product25/1
  QnL/1 -> Sum29/2
  Sum24/1 -> Sum19/3
  Integrator/1 -> WFlowTur/1, Divide3/1, Product30/2, Abs/1, Sum29/1
  Sum36/1 -> Divide5/1
  Sum34/1 -> Product26/1
  [WturErr] -> Product34/2
  Sum25/1 -> Switch7/3
  [Gate] -> 1-D Lookup Table/1
  Divide5/1 -> Sum35/2
  Product30/1 -> Product21/1
  Abs/1 -> Product30/1
  a2/1 -> Product28/1
  Sum32/1 -> Product29/1, Sum34/2
  GateMax/1 -> Sum36/1
  [PMpump] -> Switch9/3
  Product32/1 -> Gain22/1
  a0/1 -> Product36/1
  KpFpFt/1 -> Product21/2
  [WturErr] -> Sum31/1
  Switch8/1 -> Sum28/2
  Product25/1 -> Product24/1
  [RSC_Mode] -> Product32/2
  Gain21/1 -> Sum22/3
  Product35/1 -> MONx/1, Product36/2, Product37/1, Product28/2
  Switch7/1 -> Sum26/2
  Product26/1 -> Gain23/1
  [Head] -> Sum34/1
  Product27/1 -> Product28/3
  Divide3/1 -> Product31/1, Product31/2
  Product37/1 -> Sum32/2
  Saturation Dynamic/1 -> SPDref/1, [SPDref]
  Product24/1 -> Sum34/3
  KpFp/1 -> Sum35/1
  [TurbPump] -> Switch8/2
  Product28/1 -> Sum32/3
  Divide6/1 -> [G1TMECH]
  Product34/1 -> Sum30/2
  Sum29/1 -> Product33/3
  Abs1/1 -> Product37/3
  At/1 -> Product33/1
  Switch9/1 -> Divide6/1
  Constant19/1 -> Product29/3
  Constant13/1 -> Product22/1
  Constant4/1 -> Sum20/2
  Constant11/1 -> Sum19/1
  Transfer Fcn1/1 -> Saturation3/1
  Sum27/1 -> Product23/1
  Product36/1 -> Sum32/1
  wr/1 -> [wr]
  TurbPump/1 -> [TurbPump]
  RSC_Mode/1 -> [RSC_Mode]
  [G1TMECH] -> Tm_PSH/1
  [PSTATref] -> PSTATref/1
  GOVStart/1 -> [GOVStart]
  Constant1/1 -> Saturation Dynamic/3
  [RSC_Mode] -> Switch1/2
  Constant5/1 -> Switch1/1
  Constant3/1 -> Switch1/3
  Switch1/1 -> Saturation Dynamic/1
  PI Control Governor/1(TurOut) -> TurOut/1, Switch8/1
  [PSET] -> Sum20/1
  [PSET] -> Sum23/1
  Sum19/1 -> GATEref/1, [GATEref], Divide4/1
  [SPDref] -> Divide4/2
  Constant/1 -> Gain1/1
  Constant14/1 -> Gain2/1
  Gain2/1 -> Product1/1
  Gain1/1 -> Product1/2
  Product1/1 -> EMAX/1, [EMAX]
  Constant15/1 -> Product2/1
  [EMAX] -> Product2/2
  Product2/1 -> Sum1/1
  [G1TMECH] -> Gain3/1
  Gain3/1 -> Integrator3/1
  Integrator3/1 -> Sum1/2
  Sum1/1 -> Divide1/1
  [EMAX] -> Divide1/2
  Divide1/1 -> Gain4/1
  [SOC] -> Gain5/1
  Constant16/1 -> Product3/1
  Gain5/1 -> Product3/2
  Product3/1 -> Sum2/1
  Constant17/1 -> Sum2/2
  Sum2/1 -> Head/1, [Head]
  Gain4/1 -> SOC/1, [SOC]
  [SPDref] -> SPDref_out/1
  [SOC] -> SOC_out/1

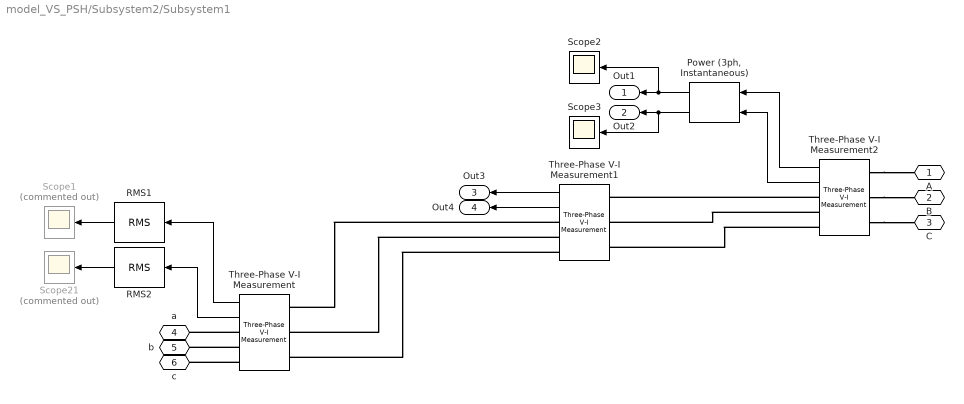
== system model_VS_PSH/Subsystem2/Subsystem1 ==
  "Power (3ph, Instantaneous)" : powerlib_meascontrol/Measurements/Power (3ph, Instantaneous)
  RMS1 : powerlib_meascontrol/Measurements/RMS  TrueRMS=off  Freq=60  RMSInit=1  Ts=Ts
  RMS2 : powerlib_meascontrol/Measurements/RMS  TrueRMS=off  Freq=60  RMSInit=1  Ts=Ts
  Scope1 : Scope  Commented=on
  Scope2 : Scope
  Scope21 : Scope  Commented=on
  Scope3 : Scope
  Three-Phase V-I Measurement : powerlib/Measurements/Three-Phase V-I Measurement  VoltageMeasurement=phase-to-phase  SetLabelV=off  LabelV=Vabc  Vpu=off  VpuLL=off  CurrentMeasurement=yes  SetLabelI=off  LabelI=Iabc  Ipu=off  Pbase=100e6  Vbase=500e3  OutputType=Complex  PhasorSimulation=off  PSBequivalent=0
  Three-Phase V-I Measurement1 : powerlib/Measurements/Three-Phase V-I Measurement  VoltageMeasurement=phase-to-ground  SetLabelV=off  LabelV=Vabc  Vpu=off  VpuLL=off  CurrentMeasurement=yes  SetLabelI=off  LabelI=Iabc  Ipu=off  Pbase=100e6  Vbase=500e3  OutputType=Complex  PhasorSimulation=off  PSBequivalent=0
  Three-Phase V-I Measurement2 : powerlib/Measurements/Three-Phase V-I Measurement  VoltageMeasurement=phase-to-ground  SetLabelV=off  LabelV=Vabc  Vpu=off  VpuLL=off  CurrentMeasurement=yes  SetLabelI=off  LabelI=Iabc  Ipu=off  Pbase=100e6  Vbase=500e3  OutputType=Complex  PhasorSimulation=off  PSBequivalent=0
  A : PMIOPort  Side=Left
  B : PMIOPort  Port=2  Side=Left
  C : PMIOPort  Port=3  Side=Left
  a : PMIOPort  Port=4  Side=Right
  b : PMIOPort  Port=5  Side=Right
  c : PMIOPort  Port=6  Side=Right
  Out1 : Outport
  Out2 : Outport  Port=2
  Out3 : Outport  Port=3
  Out4 : Outport  Port=4
  wires:
  Three-Phase V-I Measurement2/1 -> "Power (3ph, Instantaneous)"/1
  Three-Phase V-I Measurement2/2 -> "Power (3ph, Instantaneous)"/2
  "Power (3ph, Instantaneous)"/1 -> Scope2/1, Out1/1
  "Power (3ph, Instantaneous)"/2 -> Scope3/1, Out2/1
  RMS2/1 -> Scope21/1
  RMS1/1 -> Scope1/1
  Three-Phase V-I Measurement/1 -> RMS1/1
  Three-Phase V-I Measurement/2 -> RMS2/1
  Three-Phase V-I Measurement1/1 -> Out3/1
  Three-Phase V-I Measurement1/2 -> Out4/1
  connections:
  Three-Phase V-I Measurement2/RConn1 -- Three-Phase V-I Measurement1/LConn1
  Three-Phase V-I Measurement2/RConn2 -- Three-Phase V-I Measurement1/LConn2
  Three-Phase V-I Measurement2/RConn3 -- Three-Phase V-I Measurement1/LConn3
  Three-Phase V-I Measurement1/RConn2 -- Three-Phase V-I Measurement/LConn2
  Three-Phase V-I Measurement1/RConn3 -- Three-Phase V-I Measurement/LConn3
  Three-Phase V-I Measurement2/LConn1 -- A/RConn1
  Three-Phase V-I Measurement1/RConn1 -- Three-Phase V-I Measurement/LConn1
  Three-Phase V-I Measurement2/LConn2 -- B/RConn1
  Three-Phase V-I Measurement2/LConn3 -- C/RConn1
  Three-Phase V-I Measurement/RConn1 -- a/RConn1
  Three-Phase V-I Measurement/RConn2 -- b/RConn1
  Three-Phase V-I Measurement/RConn3 -- c/RConn1

== system model_VS_PSH/Subsystem2/Subsystem2 ==
  "Power (3ph, Instantaneous)" : powerlib_meascontrol/Measurements/Power (3ph, Instantaneous)
  RMS1 : powerlib_meascontrol/Measurements/RMS  TrueRMS=off  Freq=60  RMSInit=1  Ts=Ts
  RMS2 : powerlib_meascontrol/Measurements/RMS  TrueRMS=off  Freq=60  RMSInit=1  Ts=Ts
  Scope{1..3,21} (4 alike) : Scope  Commented=on
  Three-Phase V-I Measurement : powerlib/Measurements/Three-Phase V-I Measurement  VoltageMeasurement=phase-to-phase  SetLabelV=off  LabelV=Vabc  Vpu=off  VpuLL=off  CurrentMeasurement=yes  SetLabelI=off  LabelI=Iabc  Ipu=off  Pbase=100e6  Vbase=500e3  OutputType=Complex  PhasorSimulation=off  PSBequivalent=0
  Three-Phase V-I Measurement1 : powerlib/Measurements/Three-Phase V-I Measurement  VoltageMeasurement=phase-to-ground  SetLabelV=off  LabelV=Vabc  Vpu=off  VpuLL=off  CurrentMeasurement=yes  SetLabelI=off  LabelI=Iabc  Ipu=off  Pbase=100e6  Vbase=500e3  OutputType=Complex  PhasorSimulation=off  PSBequivalent=0
  Three-Phase V-I Measurement2 : powerlib/Measurements/Three-Phase V-I Measurement  VoltageMeasurement=phase-to-ground  SetLabelV=off  LabelV=Vabc  Vpu=off  VpuLL=off  CurrentMeasurement=yes  SetLabelI=off  LabelI=Iabc  Ipu=off  Pbase=100e6  Vbase=500e3  OutputType=Complex  PhasorSimulation=off  PSBequivalent=0
  A : PMIOPort  Side=Left
  B : PMIOPort  Port=2  Side=Left
  C : PMIOPort  Port=3  Side=Left
  a : PMIOPort  Port=4  Side=Right
  b : PMIOPort  Port=5  Side=Right
  c : PMIOPort  Port=6  Side=Right
  Out1 : Outport
  Out2 : Outport  Port=2
  Out3 : Outport  Port=3
  Out4 : Outport  Port=4
  wires:
  Three-Phase V-I Measurement2/1 -> "Power (3ph, Instantaneous)"/1
  Three-Phase V-I Measurement2/2 -> "Power (3ph, Instantaneous)"/2
  "Power (3ph, Instantaneous)"/1 -> Scope2/1, Out1/1
  "Power (3ph, Instantaneous)"/2 -> Scope3/1, Out2/1
  Three-Phase V-I Measurement1/1 -> Out3/1
  RMS1/1 -> Scope1/1
  Three-Phase V-I Measurement/2 -> RMS2/1
  Three-Phase V-I Measurement/1 -> RMS1/1
  RMS2/1 -> Scope21/1
  Three-Phase V-I Measurement1/2 -> Out4/1
  connections:
  Three-Phase V-I Measurement2/RConn1 -- Three-Phase V-I Measurement1/LConn1
  Three-Phase V-I Measurement2/RConn2 -- Three-Phase V-I Measurement1/LConn2
  Three-Phase V-I Measurement2/RConn3 -- Three-Phase V-I Measurement1/LConn3
  Three-Phase V-I Measurement1/RConn2 -- Three-Phase V-I Measurement/LConn2
  Three-Phase V-I Measurement1/RConn3 -- Three-Phase V-I Measurement/LConn3
  Three-Phase V-I Measurement2/LConn1 -- A/RConn1
  Three-Phase V-I Measurement1/RConn1 -- Three-Phase V-I Measurement/LConn1
  Three-Phase V-I Measurement2/LConn2 -- B/RConn1
  Three-Phase V-I Measurement2/LConn3 -- C/RConn1
  Three-Phase V-I Measurement/RConn1 -- a/RConn1
  Three-Phase V-I Measurement/RConn2 -- b/RConn1
  Three-Phase V-I Measurement/RConn3 -- c/RConn1

== system model_VS_PSH/Subsystem2/Subsystem3 ==
  "Power (3ph, Instantaneous)" : powerlib_meascontrol/Measurements/Power (3ph, Instantaneous)
  RMS1 : powerlib_meascontrol/Measurements/RMS  TrueRMS=off  Freq=60  RMSInit=1  Ts=Ts
  RMS2 : powerlib_meascontrol/Measurements/RMS  TrueRMS=off  Freq=60  RMSInit=1  Ts=Ts
  Scope1 : Scope  Commented=on
  Scope2 : Scope
  Scope21 : Scope  Commented=on
  Scope3 : Scope
  Three-Phase V-I Measurement : powerlib/Measurements/Three-Phase V-I Measurement  VoltageMeasurement=phase-to-phase  SetLabelV=off  LabelV=Vabc  Vpu=off  VpuLL=off  CurrentMeasurement=yes  SetLabelI=off  LabelI=Iabc  Ipu=off  Pbase=100e6  Vbase=500e3  OutputType=Complex  PhasorSimulation=off  PSBequivalent=0
  Three-Phase V-I Measurement1 : powerlib/Measurements/Three-Phase V-I Measurement  VoltageMeasurement=phase-to-ground  SetLabelV=off  LabelV=Vabc  Vpu=off  VpuLL=off  CurrentMeasurement=yes  SetLabelI=off  LabelI=Iabc  Ipu=off  Pbase=100e6  Vbase=500e3  OutputType=Complex  PhasorSimulation=off  PSBequivalent=0
  Three-Phase V-I Measurement2 : powerlib/Measurements/Three-Phase V-I Measurement  VoltageMeasurement=phase-to-ground  SetLabelV=off  LabelV=Vabc  Vpu=off  VpuLL=off  CurrentMeasurement=yes  SetLabelI=off  LabelI=Iabc  Ipu=off  Pbase=100e6  Vbase=500e3  OutputType=Complex  PhasorSimulation=off  PSBequivalent=0
  a : PMIOPort  Side=Right
  A : PMIOPort  Port=2  Side=Left
  b : PMIOPort  Port=3  Side=Right
  B : PMIOPort  Port=4  Side=Left
  c : PMIOPort  Port=5  Side=Right
  C : PMIOPort  Port=6  Side=Left
  Out1 : Outport
  Out2 : Outport  Port=2
  Out3 : Outport  Port=3
  Out4 : Outport  Port=4
  wires:
  Three-Phase V-I Measurement2/1 -> "Power (3ph, Instantaneous)"/1
  Three-Phase V-I Measurement2/2 -> "Power (3ph, Instantaneous)"/2
  "Power (3ph, Instantaneous)"/1 -> Scope2/1, Out1/1
  "Power (3ph, Instantaneous)"/2 -> Scope3/1, Out2/1
  RMS2/1 -> Scope21/1
  Three-Phase V-I Measurement/1 -> RMS1/1
  RMS1/1 -> Scope1/1
  Three-Phase V-I Measurement/2 -> RMS2/1
  Three-Phase V-I Measurement1/1 -> Out3/1
  Three-Phase V-I Measurement1/2 -> Out4/1
  connections:
  Three-Phase V-I Measurement2/RConn1 -- Three-Phase V-I Measurement1/LConn1
  Three-Phase V-I Measurement2/RConn2 -- Three-Phase V-I Measurement1/LConn2
  Three-Phase V-I Measurement2/RConn3 -- Three-Phase V-I Measurement1/LConn3
  Three-Phase V-I Measurement2/LConn1 -- A/RConn1
  Three-Phase V-I Measurement2/LConn2 -- B/RConn1
  Three-Phase V-I Measurement2/LConn3 -- C/RConn1
  Three-Phase V-I Measurement1/RConn1 -- Three-Phase V-I Measurement/LConn1
  Three-Phase V-I Measurement1/RConn2 -- Three-Phase V-I Measurement/LConn2
  Three-Phase V-I Measurement1/RConn3 -- Three-Phase V-I Measurement/LConn3
  Three-Phase V-I Measurement/RConn1 -- a/RConn1
  Three-Phase V-I Measurement/RConn2 -- b/RConn1
  Three-Phase V-I Measurement/RConn3 -- c/RConn1

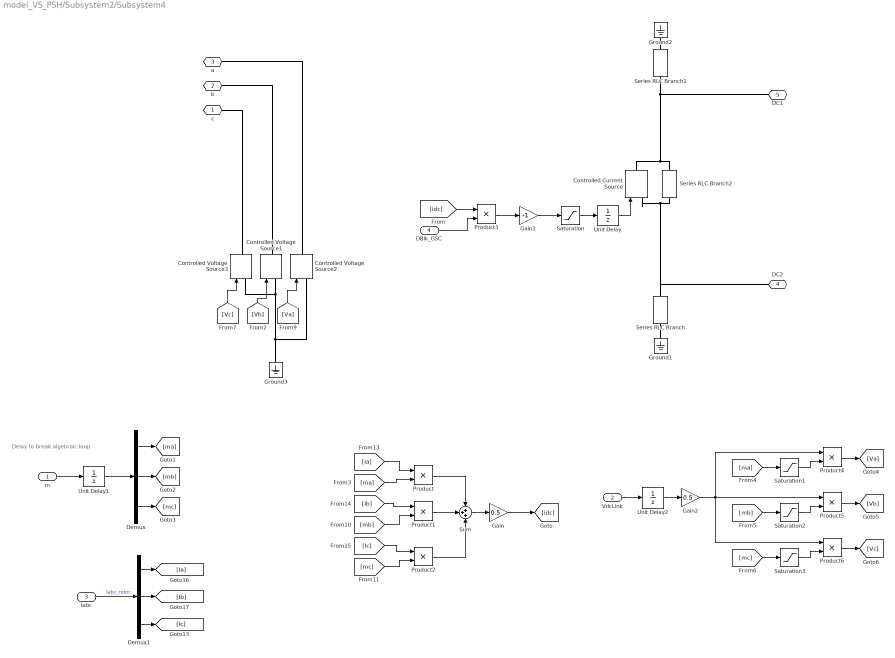
== system model_VS_PSH/Subsystem2/Subsystem4 ==
  note: Delay to break algebraic loop
  m : Inport
  VdcLink : Inport  Port=2
  Iabc : Inport  Port=3
  DBlk_GSC : Inport  Port=4
  Controlled Current Source : powerlib/Electrical Sources/Controlled Current Source  Initialize=on  Source_Type=AC  Amplitude=0  Phase=0  Frequency=0  Measurements=None
  Controlled Voltage Source1 : powerlib/Electrical Sources/Controlled Voltage Source  Initialize=on  Source_Type=AC  Amplitude=0  Phase=0  Frequency=0  Measurements=None
  Controlled Voltage Source2 : powerlib/Electrical Sources/Controlled Voltage Source  Initialize=on  Source_Type=AC  Amplitude=0  Phase=0  Frequency=0  Measurements=None
  Controlled Voltage Source3 : powerlib/Electrical Sources/Controlled Voltage Source  Initialize=on  Source_Type=AC  Amplitude=0  Phase=0  Frequency=0  Measurements=None
  Demux : Demux  Outputs=3
  Demux1 : Demux  Outputs=3
  Gain : Gain  Gain=0.5
  Gain1 : Gain  Gain=-1
  Gain2 : Gain  Gain=0.5
  Ground1 : powerlib/Elements/Ground  LConnTagsString=a
  Ground2 : powerlib/Elements/Ground  LConnTagsString=a
  Ground3 : powerlib/Elements/Ground  LConnTagsString=a
  Product{,1..6} (7 alike) : Product
  Saturation : Saturate  UpperLimit=1e10  LowerLimit=-1e10
  Saturation1 : Saturate  UpperLimit=1  LowerLimit=-1
  Saturation2 : Saturate  UpperLimit=1  LowerLimit=-1
  Saturation3 : Saturate  UpperLimit=1  LowerLimit=-1
  Series RLC Branch : powerlib/Elements/Series RLC Branch  LConnTagsString=__new0  RConnTagsString=__new0  BranchType=R  Resistance=1e6  Inductance=1e-3  SetiL0=off  InitialCurrent=0  Capacitance=1e-6  Setx0=off  InitialVoltage=0  Measurements=None
  Series RLC Branch1 : powerlib/Elements/Series RLC Branch  LConnTagsString=__new0  RConnTagsString=__new0  BranchType=R  Resistance=1e6  Inductance=1e-3  SetiL0=off  InitialCurrent=0  Capacitance=1e-6  Setx0=off  InitialVoltage=0  Measurements=None
  Series RLC Branch2 : powerlib/Elements/Series RLC Branch  LConnTagsString=__new0  RConnTagsString=__new0  BranchType=R  Resistance=1e6  Inductance=1e-3  SetiL0=off  InitialCurrent=0  Capacitance=1e-6  Setx0=off  InitialVoltage=0  Measurements=None
  Sum : Sum  Inputs=+++
  Unit Delay : UnitDelay  SampleTime=-1  HasFrameUpgradeWarning=on
  Unit Delay1 : UnitDelay  SampleTime=-1  HasFrameUpgradeWarning=on
  Unit Delay2 : UnitDelay  SampleTime=-1  HasFrameUpgradeWarning=on
  c : PMIOPort  Side=Left
  b : PMIOPort  Port=2  Side=Left
  a : PMIOPort  Port=3  Side=Left
  DC2 : PMIOPort  Port=4  Side=Right
  DC1 : PMIOPort  Port=5  Side=Right
  wires:
  [Vb] -> Controlled Voltage Source1/1
  [Va] -> Controlled Voltage Source2/1
  [Ib] -> Product1/1
  Product6/1 -> [Vc]
  [ma] -> Saturation1/1
  [mc] -> Product2/2
  Product/1 -> Sum/1
  [Ic] -> Product2/1
  Saturation3/1 -> Product6/2
  [Vc] -> Controlled Voltage Source3/1
  Saturation2/1 -> Product5/2
  [mb] -> Product1/2
  Product4/1 -> [Va]
  Gain1/1 -> Saturation/1
  [Ia] -> Product/1
  [mc] -> Saturation3/1
  Product1/1 -> Sum/2
  [mb] -> Saturation2/1
  Saturation1/1 -> Product4/2
  [ma] -> Product/2
  Product2/1 -> Sum/3
  Product5/1 -> [Vb]
  Gain2/1 -> Product6/1, Product4/1, Product5/1
  Gain/1 -> [idc]
  Sum/1 -> Gain/1
  Demux/1 -> [ma]
  Demux/2 -> [mb]
  Demux/3 -> [mc]
  Demux1/2 -> [Ib]
  Demux1/1 -> [Ia]
  Iabc/1 -> Demux1/1  "Iabc_rotor"
  Demux1/3 -> [Ic]
  DBlk_GSC/1 -> Product3/2
  [idc] -> Product3/1
  Product3/1 -> Gain1/1
  m/1 -> Unit Delay1/1
  Unit Delay1/1 -> Demux/1
  Saturation/1 -> Unit Delay/1
  Unit Delay/1 -> Controlled Current Source/1
  VdcLink/1 -> Unit Delay2/1
  Unit Delay2/1 -> Gain2/1
  connections:
  Controlled Voltage Source2/RConn1 -- a/RConn1
  Controlled Voltage Source3/RConn1 -- c/RConn1
  DC1/RConn1 -- Series RLC Branch1/RConn1 -- Controlled Current Source/RConn1 -- Series RLC Branch2/LConn1
  Series RLC Branch/LConn1 -- DC2/RConn1 -- Controlled Current Source/LConn1 -- Series RLC Branch2/RConn1
  Controlled Voltage Source1/LConn1 -- Controlled Voltage Source3/LConn1 -- Ground3/LConn1 -- Controlled Voltage Source2/LConn1
  Controlled Voltage Source1/RConn1 -- b/RConn1
  Series RLC Branch/RConn1 -- Ground1/LConn1
  Series RLC Branch1/LConn1 -- Ground2/LConn1
